simulink model "REFvsFI"  (R2023a)
settings: Solver=FixedStepAuto  StartTime=0.0  StopTime=T  RelTol=1e-3  EnableMultiTasking=on
values from neighbouring files (symbols this model uses):
  Ts = 1    [TestDataGen.m]
libraries: My_FI_Operations x114, simulink x2
(part 5 of 5)

== system REFvsFI/ref model/multb0_1 ==
  In2 : Inport
  In1 : Inport  Port=2
  Product : Product  OutDataTypeStr=double  RndMeth=Nearest
  Out1 : Outport
  wires:
  In2/1 -> Product/2
  Product/1 -> Out1/1
  In1/1 -> Product/1

== system REFvsFI/ref model/multb0_2 ==
  In2 : Inport
  In1 : Inport  Port=2
  Product : Product  OutDataTypeStr=double  RndMeth=Nearest
  Out1 : Outport
  wires:
  In2/1 -> Product/2
  Product/1 -> Out1/1
  In1/1 -> Product/1

== system REFvsFI/ref model/multb0_3 ==
  In2 : Inport
  In1 : Inport  Port=2
  Product : Product  OutDataTypeStr=double  RndMeth=Nearest
  Out1 : Outport
  wires:
  In2/1 -> Product/2
  Product/1 -> Out1/1
  In1/1 -> Product/1

== system REFvsFI/ref model/multb10_1 ==
  In2 : Inport
  In1 : Inport  Port=2
  Product : Product  OutDataTypeStr=double  RndMeth=Nearest
  Out1 : Outport
  wires:
  Product/1 -> Out1/1
  In1/1 -> Product/1
  In2/1 -> Product/2

== system REFvsFI/ref model/multb10_2 ==
  In2 : Inport
  In1 : Inport  Port=2
  Product : Product  OutDataTypeStr=double  RndMeth=Nearest
  Out1 : Outport
  wires:
  Product/1 -> Out1/1
  In1/1 -> Product/1
  In2/1 -> Product/2

== system REFvsFI/ref model/multb10_3 ==
  In2 : Inport
  In1 : Inport  Port=2
  Product : Product  OutDataTypeStr=double  RndMeth=Nearest
  Out1 : Outport
  wires:
  Product/1 -> Out1/1
  In1/1 -> Product/1
  In2/1 -> Product/2

== system REFvsFI/ref model/multb12_1 ==
  In2 : Inport
  In1 : Inport  Port=2
  Product : Product  OutDataTypeStr=double  RndMeth=Nearest
  Out1 : Outport
  wires:
  Product/1 -> Out1/1
  In1/1 -> Product/1
  In2/1 -> Product/2

== system REFvsFI/ref model/multb12_2 ==
  In2 : Inport
  In1 : Inport  Port=2
  Product : Product  OutDataTypeStr=double  RndMeth=Nearest
  Out1 : Outport
  wires:
  Product/1 -> Out1/1
  In1/1 -> Product/1
  In2/1 -> Product/2

== system REFvsFI/ref model/multb12_3 ==
  In2 : Inport
  In1 : Inport  Port=2
  Product : Product  OutDataTypeStr=double  RndMeth=Nearest
  Out1 : Outport
  wires:
  Product/1 -> Out1/1
  In1/1 -> Product/1
  In2/1 -> Product/2

== system REFvsFI/ref model/multb2_1 ==
  In2 : Inport
  In1 : Inport  Port=2
  Product : Product  OutDataTypeStr=double  RndMeth=Nearest
  Out1 : Outport
  wires:
  In1/1 -> Product/1
  In2/1 -> Product/2
  Product/1 -> Out1/1

== system REFvsFI/ref model/multb2_2 ==
  In2 : Inport
  In1 : Inport  Port=2
  Product : Product  OutDataTypeStr=double  RndMeth=Nearest
  Out1 : Outport
  wires:
  In1/1 -> Product/1
  In2/1 -> Product/2
  Product/1 -> Out1/1

== system REFvsFI/ref model/multb2_3 ==
  In2 : Inport
  In1 : Inport  Port=2
  Product : Product  OutDataTypeStr=double  RndMeth=Nearest
  Out1 : Outport
  wires:
  In1/1 -> Product/1
  In2/1 -> Product/2
  Product/1 -> Out1/1

== system REFvsFI/ref model/multb4_1 ==
  In2 : Inport
  In1 : Inport  Port=2
  Product : Product  OutDataTypeStr=double  RndMeth=Nearest
  Out1 : Outport
  wires:
  In2/1 -> Product/2
  In1/1 -> Product/1
  Product/1 -> Out1/1

== system REFvsFI/ref model/multb4_2 ==
  In2 : Inport
  In1 : Inport  Port=2
  Product : Product  OutDataTypeStr=double  RndMeth=Nearest
  Out1 : Outport
  wires:
  In2/1 -> Product/2
  In1/1 -> Product/1
  Product/1 -> Out1/1

== system REFvsFI/ref model/multb4_3 ==
  In2 : Inport
  In1 : Inport  Port=2
  Product : Product  OutDataTypeStr=double  RndMeth=Nearest
  Out1 : Outport
  wires:
  In2/1 -> Product/2
  In1/1 -> Product/1
  Product/1 -> Out1/1

== system REFvsFI/ref model/multb6_1 ==
  In2 : Inport
  In1 : Inport  Port=2
  Product : Product  OutDataTypeStr=double  RndMeth=Nearest
  Out1 : Outport
  wires:
  In2/1 -> Product/2
  Product/1 -> Out1/1
  In1/1 -> Product/1

== system REFvsFI/ref model/multb6_2 ==
  In2 : Inport
  In1 : Inport  Port=2
  Product : Product  OutDataTypeStr=double  RndMeth=Nearest
  Out1 : Outport
  wires:
  In2/1 -> Product/2
  Product/1 -> Out1/1
  In1/1 -> Product/1

== system REFvsFI/ref model/multb6_3 ==
  In2 : Inport
  In1 : Inport  Port=2
  Product : Product  OutDataTypeStr=double  RndMeth=Nearest
  Out1 : Outport
  wires:
  In2/1 -> Product/2
  Product/1 -> Out1/1
  In1/1 -> Product/1

== system REFvsFI/ref model/multb8_1 ==
  In2 : Inport
  In1 : Inport  Port=2
  Product : Product  OutDataTypeStr=double  RndMeth=Nearest
  Out1 : Outport
  wires:
  Product/1 -> Out1/1
  In1/1 -> Product/1
  In2/1 -> Product/2

== system REFvsFI/ref model/multb8_2 ==
  In2 : Inport
  In1 : Inport  Port=2
  Product : Product  OutDataTypeStr=double  RndMeth=Nearest
  Out1 : Outport
  wires:
  Product/1 -> Out1/1
  In1/1 -> Product/1
  In2/1 -> Product/2

== system REFvsFI/ref model/multb8_3 ==
  In2 : Inport
  In1 : Inport  Port=2
  Product : Product  OutDataTypeStr=double  RndMeth=Nearest
  Out1 : Outport
  wires:
  Product/1 -> Out1/1
  In1/1 -> Product/1
  In2/1 -> Product/2

== system REFvsFI/ref model/suma2_1 ==
  In2 : Inport
  In1 : Inport  Port=2
  Add : Sum  OutDataTypeStr=double  RndMeth=Nearest
  Out1 : Outport
  wires:
  In1/1 -> Add/1
  Add/1 -> Out1/1
  In2/1 -> Add/2

== system REFvsFI/ref model/suma2_2 ==
  In2 : Inport
  In1 : Inport  Port=2
  Add : Sum  OutDataTypeStr=double  RndMeth=Nearest
  Out1 : Outport
  wires:
  In1/1 -> Add/1
  Add/1 -> Out1/1
  In2/1 -> Add/2

== system REFvsFI/ref model/suma2_3 ==
  In2 : Inport
  In1 : Inport  Port=2
  Add : Sum  OutDataTypeStr=double  RndMeth=Nearest
  Out1 : Outport
  wires:
  In1/1 -> Add/1
  Add/1 -> Out1/1
  In2/1 -> Add/2

== system REFvsFI/ref model/suma4_1 ==
  In1 : Inport
  In2 : Inport  Port=2
  Add : Sum  OutDataTypeStr=double  RndMeth=Nearest
  Out1 : Outport
  wires:
  In1/1 -> Add/1
  In2/1 -> Add/2
  Add/1 -> Out1/1

== system REFvsFI/ref model/suma4_2 ==
  In1 : Inport
  In2 : Inport  Port=2
  Add : Sum  OutDataTypeStr=double  RndMeth=Nearest
  Out1 : Outport
  wires:
  In1/1 -> Add/1
  In2/1 -> Add/2
  Add/1 -> Out1/1

== system REFvsFI/ref model/suma4_3 ==
  In1 : Inport
  In2 : Inport  Port=2
  Add : Sum  OutDataTypeStr=double  RndMeth=Nearest
  Out1 : Outport
  wires:
  In1/1 -> Add/1
  In2/1 -> Add/2
  Add/1 -> Out1/1

== system REFvsFI/ref model/suma6_1 ==
  In1 : Inport
  In2 : Inport  Port=2
  Add : Sum  OutDataTypeStr=double  RndMeth=Nearest
  Out1 : Outport
  wires:
  Add/1 -> Out1/1
  In2/1 -> Add/2
  In1/1 -> Add/1

== system REFvsFI/ref model/suma6_2 ==
  In1 : Inport
  In2 : Inport  Port=2
  Add : Sum  OutDataTypeStr=double  RndMeth=Nearest
  Out1 : Outport
  wires:
  Add/1 -> Out1/1
  In2/1 -> Add/2
  In1/1 -> Add/1

== system REFvsFI/ref model/suma6_3 ==
  In1 : Inport
  In2 : Inport  Port=2
  Add : Sum  OutDataTypeStr=double  RndMeth=Nearest
  Out1 : Outport
  wires:
  Add/1 -> Out1/1
  In2/1 -> Add/2
  In1/1 -> Add/1

== system REFvsFI/ref model/sumb10_1 ==
  In2 : Inport
  In1 : Inport  Port=2
  Add : Sum  OutDataTypeStr=double  RndMeth=Nearest
  Out1 : Outport
  wires:
  Add/1 -> Out1/1
  In2/1 -> Add/2
  In1/1 -> Add/1

== system REFvsFI/ref model/sumb10_2 ==
  In2 : Inport
  In1 : Inport  Port=2
  Add : Sum  OutDataTypeStr=double  RndMeth=Nearest
  Out1 : Outport
  wires:
  Add/1 -> Out1/1
  In2/1 -> Add/2
  In1/1 -> Add/1

== system REFvsFI/ref model/sumb10_3 ==
  In2 : Inport
  In1 : Inport  Port=2
  Add : Sum  OutDataTypeStr=double  RndMeth=Nearest
  Out1 : Outport
  wires:
  Add/1 -> Out1/1
  In2/1 -> Add/2
  In1/1 -> Add/1

== system REFvsFI/ref model/sumb12_1 ==
  In2 : Inport
  In1 : Inport  Port=2
  Add : Sum
  Out1 : Outport
  wires:
  In2/1 -> Add/2
  Add/1 -> Out1/1
  In1/1 -> Add/1

== system REFvsFI/ref model/sumb12_2 ==
  In2 : Inport
  In1 : Inport  Port=2
  Add : Sum
  Out1 : Outport
  wires:
  In2/1 -> Add/2
  Add/1 -> Out1/1
  In1/1 -> Add/1

== system REFvsFI/ref model/sumb12_3 ==
  In2 : Inport
  In1 : Inport  Port=2
  Add : Sum
  Out1 : Outport
  wires:
  In2/1 -> Add/2
  Add/1 -> Out1/1
  In1/1 -> Add/1

== system REFvsFI/ref model/sumb2_1 ==
  In2 : Inport
  In1 : Inport  Port=2
  Add : Sum  OutDataTypeStr=double  RndMeth=Nearest
  Out1 : Outport
  wires:
  Add/1 -> Out1/1
  In2/1 -> Add/2
  In1/1 -> Add/1

== system REFvsFI/ref model/sumb2_2 ==
  In2 : Inport
  In1 : Inport  Port=2
  Add : Sum  OutDataTypeStr=double  RndMeth=Nearest
  Out1 : Outport
  wires:
  Add/1 -> Out1/1
  In2/1 -> Add/2
  In1/1 -> Add/1

== system REFvsFI/ref model/sumb2_3 ==
  In2 : Inport
  In1 : Inport  Port=2
  Add : Sum  OutDataTypeStr=double  RndMeth=Nearest
  Out1 : Outport
  wires:
  Add/1 -> Out1/1
  In2/1 -> Add/2
  In1/1 -> Add/1

== system REFvsFI/ref model/sumb4_1 ==
  In2 : Inport
  In1 : Inport  Port=2
  Add : Sum  OutDataTypeStr=double  RndMeth=Nearest
  Out1 : Outport
  wires:
  Add/1 -> Out1/1
  In2/1 -> Add/2
  In1/1 -> Add/1

== system REFvsFI/ref model/sumb4_2 ==
  In2 : Inport
  In1 : Inport  Port=2
  Add : Sum  OutDataTypeStr=double  RndMeth=Nearest
  Out1 : Outport
  wires:
  Add/1 -> Out1/1
  In2/1 -> Add/2
  In1/1 -> Add/1

== system REFvsFI/ref model/sumb4_3 ==
  In2 : Inport
  In1 : Inport  Port=2
  Add : Sum  OutDataTypeStr=double  RndMeth=Nearest
  Out1 : Outport
  wires:
  Add/1 -> Out1/1
  In2/1 -> Add/2
  In1/1 -> Add/1

== system REFvsFI/ref model/sumb6_1 ==
  In2 : Inport
  In1 : Inport  Port=2
  Add : Sum  OutDataTypeStr=double  RndMeth=Nearest
  Out1 : Outport
  wires:
  In2/1 -> Add/2
  In1/1 -> Add/1
  Add/1 -> Out1/1

== system REFvsFI/ref model/sumb6_2 ==
  In2 : Inport
  In1 : Inport  Port=2
  Add : Sum  OutDataTypeStr=double  RndMeth=Nearest
  Out1 : Outport
  wires:
  In2/1 -> Add/2
  In1/1 -> Add/1
  Add/1 -> Out1/1

== system REFvsFI/ref model/sumb6_3 ==
  In2 : Inport
  In1 : Inport  Port=2
  Add : Sum  OutDataTypeStr=double  RndMeth=Nearest
  Out1 : Outport
  wires:
  In2/1 -> Add/2
  In1/1 -> Add/1
  Add/1 -> Out1/1

== system REFvsFI/ref model/sumb8_1 ==
  In2 : Inport
  In1 : Inport  Port=2
  Add : Sum  OutDataTypeStr=double  RndMeth=Nearest
  Out1 : Outport
  wires:
  In2/1 -> Add/2
  In1/1 -> Add/1
  Add/1 -> Out1/1

== system REFvsFI/ref model/sumb8_2 ==
  In2 : Inport
  In1 : Inport  Port=2
  Add : Sum  OutDataTypeStr=double  RndMeth=Nearest
  Out1 : Outport
  wires:
  In2/1 -> Add/2
  In1/1 -> Add/1
  Add/1 -> Out1/1

== system REFvsFI/ref model/sumb8_3 ==
  In2 : Inport
  In1 : Inport  Port=2
  Add : Sum  OutDataTypeStr=double  RndMeth=Nearest
  Out1 : Outport
  wires:
  In2/1 -> Add/2
  In1/1 -> Add/1
  Add/1 -> Out1/1

== system REFvsFI/ref model/sumd-2 ==
  In1 : Inport
  In2 : Inport  Port=2
  Add : Sum  OutDataTypeStr=double  RndMeth=Nearest
  Out1 : Outport
  wires:
  In1/1 -> Add/1
  Add/1 -> Out1/1
  In2/1 -> Add/2

== system REFvsFI/ref model/sumd-3 ==
  In1 : Inport
  In2 : Inport  Port=2
  Add : Sum  OutDataTypeStr=double  RndMeth=Nearest
  Out1 : Outport
  wires:
  In1/1 -> Add/1
  Add/1 -> Out1/1
  In2/1 -> Add/2

== system REFvsFI/ref model/sumd-4 ==
  In1 : Inport
  In2 : Inport  Port=2
  Add : Sum  OutDataTypeStr=double  RndMeth=Nearest
  Out1 : Outport
  wires:
  In2/1 -> Add/2
  In1/1 -> Add/1
  Add/1 -> Out1/1

== system REFvsFI/ref model/sumin_1 ==
  In1 : Inport
  In2 : Inport  Port=2
  Add : Sum  OutDataTypeStr=double  RndMeth=Nearest
  Out1 : Outport
  wires:
  Add/1 -> Out1/1
  In1/1 -> Add/1
  In2/1 -> Add/2

== system REFvsFI/ref model/sumin_2 ==
  In1 : Inport
  In2 : Inport  Port=2
  Add : Sum  OutDataTypeStr=double  RndMeth=Nearest
  Out1 : Outport
  wires:
  Add/1 -> Out1/1
  In1/1 -> Add/1
  In2/1 -> Add/2

== system REFvsFI/ref model/sumin_3 ==
  In1 : Inport
  In2 : Inport  Port=2
  Add : Sum  OutDataTypeStr=double  RndMeth=Nearest
  Out1 : Outport
  wires:
  Add/1 -> Out1/1
  In1/1 -> Add/1
  In2/1 -> Add/2

== system REFvsFI/ref model/sumq-1 ==
  In2 : Inport
  In1 : Inport  Port=2
  Add : Sum  OutDataTypeStr=double  RndMeth=Nearest
  Out1 : Outport
  wires:
  In1/1 -> Add/1
  In2/1 -> Add/2
  Add/1 -> Out1/1

== system REFvsFI/ref model/sumq-2 ==
  In1 : Inport
  In2 : Inport  Port=2
  Add : Sum  OutDataTypeStr=double  RndMeth=Nearest
  Out1 : Outport
  wires:
  Add/1 -> Out1/1
  In1/1 -> Add/1
  In2/1 -> Add/2

== system REFvsFI/ref model/sumq-3 ==
  In1 : Inport
  In2 : Inport  Port=2
  Add : Sum  OutDataTypeStr=double  RndMeth=Nearest
  Out1 : Outport
  wires:
  In2/1 -> Add/2
  Add/1 -> Out1/1
  In1/1 -> Add/1
